simulink model "test03"  (R2021a)
settings: Solver=VariableStepAuto  StartTime=0.0  StopTime=10  RelTol=1e-3
values from neighbouring files (symbols this model uses):
  cic = climate_ic    [test03_script.m]
  params = climate_p    [test03_script.m]
libraries: HORTISIM x8
settings Model: Creator=djoroya  LastModifiedBy=djoroya
settings DebuggingCC: UnconnectedInputMsg=none  UnconnectedOutputMsg=none  UnconnectedLineMsg=none

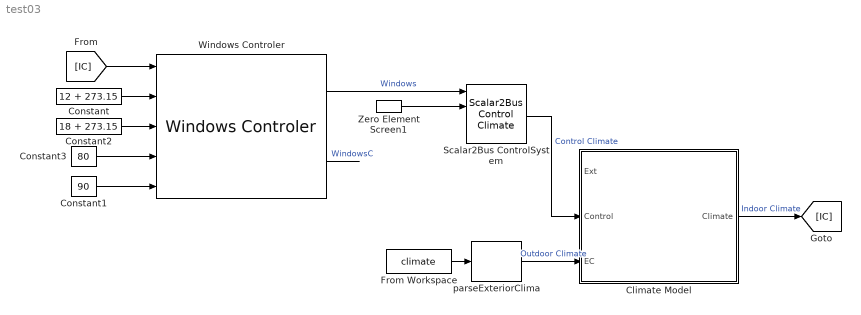
== system test03 ==
  Climate Model : Subsystem  AncestorBlock=HORTISIM/Climate/Models/Climate Model  mask{params=params, x0=cic}
      mask Display: image('$imagefile'); % Use "Edit Image" on toolstrip to change.
  Constant : Constant  Value=12 + 273.15
  Constant1 : Constant  Value=90
  Constant2 : Constant  Value=18 + 273.15
  Constant3 : Constant  Value=80
  From Workspace : FromWorkspace  VariableName=climate
  Scalar2Bus ControlSystem : HORTISIM/Other  Functions/Scalar2Bus  Control Climate  SystemSampleTime=-1  VariantActivationTime=update diagram  Latency=0  AutoFrameSizeCalculation=off
      settings: SourceProductName=Horti Simulator
  Windows Controler : HORTISIM/Climate/Controls/Windows Controler  params=win_p
      settings: SourceProductName=Horti Simulator
  Zero Element Screen1 : HORTISIM/Other  Functions/Zero Element Screen  SystemSampleTime=-1  VariantActivationTime=update diagram  Latency=0  AutoFrameSizeCalculation=off
      settings: SourceProductName=Horti Simulator
  parseExteriorClima : HORTISIM/Other  Functions/parseExteriorClima  SystemSampleTime=-1  VariantActivationTime=update diagram  Latency=0  AutoFrameSizeCalculation=off
      settings: SourceProductName=Horti Simulator
  wires:
  From Workspace/1 -> parseExteriorClima/1
  parseExteriorClima/1 -> Climate Model/3(EC)  "Outdoor Climate"
  Climate Model/1(Climate) -> [IC]  "Indoor Climate"
  Scalar2Bus ControlSystem/1 -> Climate Model/2(Control)  "Control Climate"
  Windows Controler/1 -> Scalar2Bus ControlSystem/1  "Windows"
  [IC] -> Windows Controler/1
  Constant/1 -> Windows Controler/2
  Constant2/1 -> Windows Controler/3
  Constant3/1 -> Windows Controler/4
  Constant1/1 -> Windows Controler/5
  Windows Controler/2 -> ?  "WindowsC"
  Zero Element Screen1/1 -> Scalar2Bus ControlSystem/2

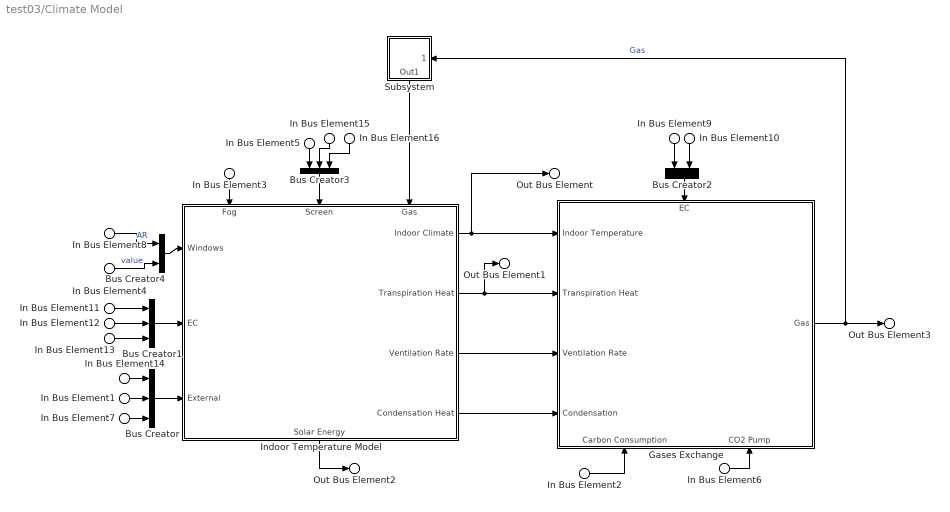
== system test03/Climate Model ==
  In Bus Element14 : Inport  PortName=Ext  Element=QT
  In Bus Element1 : Inport  PortName=Ext  Element=QV
  In Bus Element2 : Inport  PortName=Ext  Element=CC
  In Bus Element7 : Inport  PortName=Ext  Element=A
  In Bus Element3 : Inport  Port=2  PortName=Control  Element=Fog
  In Bus Element5 : Inport  Port=2  PortName=Control  Element=Screen.gamma_max
  In Bus Element15 : Inport  Port=2  PortName=Control  Element=Screen.value
  In Bus Element16 : Inport  Port=2  PortName=Control  Element=Screen.beta
  In Bus Element6 : Inport  Port=2  PortName=Control  Element=CO2
  In Bus Element8 : Inport  Port=2  PortName=Control  Element=Windows.AR
  In Bus Element4 : Inport  Port=2  PortName=Control  Element=Windows.value
  In Bus Element9 : Inport  Port=3  PortName=EC  Element=HR
  In Bus Element10 : Inport  Port=3  PortName=EC  Element=Temp
  In Bus Element11 : Inport  Port=3  PortName=EC  Element=Temp
  In Bus Element12 : Inport  Port=3  PortName=EC  Element=Rad
  In Bus Element13 : Inport  Port=3  PortName=EC  Element=Wind
  Bus Creator : BusCreator  Inputs=3
  Bus Creator1 : BusCreator  Inputs=3
  Bus Creator2 : BusCreator  Inputs=2
  Bus Creator3 : BusCreator  Inputs=3
  Bus Creator4 : BusCreator  Inputs=2
  Gases Exchange : Subsystem
      settings: PortSchema="{\"entries\":[{\"content\":{\"sides\":[{\"content\":{\"connectorIds\":[\"In1\",\"In2\",\"In3\",\"In4\"]},\"type\":\"ConnectorPlacement.EquallySpacedRectSide\",\"uuid\":\"550da9a1-5f22-4db3-9ee3-e3750278f626\"},{\"content\":{\"connectorIds\":[\"Out1\"],\"side\":\"RIGHT\"},\"type\":\"ConnectorPlacement.EquallySpacedRectSide\",\"uuid\":\"cf559ec0-337d-42e7-96bb-a49ff9e682f6\"},{\"content\":{\"connectorIds\":[\"In5\"],\"side\":\"TOP\"},\"type\":\"ConnectorPlacement.EquallySpacedRectSide\",\"uuid\":\"d9874986-c35c-443c-9325-7a886074565b\"},{\"content\":{\"connectorIds\":[\"In6\",\"In7\"],\"side\":\"BOTTOM\"},\"type\":\"ConnectorPlacement.EquallySpacedRectSide\",\"uuid\":\"7f205c84-db2c-43a4-94ce-a6d2142a4e50\"}]},\"type\":\"ConnectorPlacement.EquallySpacedConnector\",\"uuid\":\"56c5cbc1-f580-43fc-9d79-62500ce9be4b\"}],\"packageUris\":[\"http://schema.mathworks.com/mf0/Connector/R2020b\"],\"version\":\"1.0\"}"
  Indoor Temperature Model : Subsystem
      settings: PortSchema="{\"entries\":[{\"content\":{\"sides\":[{\"content\":{\"connectorIds\":[\"In1\",\"In2\",\"In3\"]},\"type\":\"ConnectorPlacement.EquallySpacedRectSide\",\"uuid\":\"402556d7-b277-4cb3-8556-883bae99c69c\"},{\"content\":{\"connectorIds\":[\"Out1\",\"Out2\",\"Out3\",\"Out4\"],\"side\":\"RIGHT\"},\"type\":\"ConnectorPlacement.EquallySpacedRectSide\",\"uuid\":\"e8ec9f82-8759-4d98-a5e5-ef4db996ec8c\"},{\"content\":{\"connectorIds\":[\"In4\",\"In5\",\"In6\"],\"side\":\"TOP\"},\"type\":\"ConnectorPlacement.EquallySpacedRectSide\",\"uuid\":\"99d33cea-a089-4bcb-9505-68914c63f152\"},{\"content\":{\"connectorIds\":[\"Out5\"],\"side\":\"BOTTOM\"},\"type\":\"ConnectorPlacement.EquallySpacedRectSide\",\"uuid\":\"61ead6b3-0464-47f9-9f23-19f86056b325\"}]},\"type\":\"ConnectorPlacement.EquallySpacedConnector\",\"uuid\":\"a07dfd2f-7b40-4439-87f5-f093ac984b26\"}],\"packageUris\":[\"http://schema.mathworks.com/mf0/Connector/R2020b\"],\"version\":\"1.0\"}"
  Subsystem : Subsystem
      settings: PortSchema="{\"entries\":[{\"content\":{\"sides\":[{\"content\":{\"connectorIds\":[]},\"type\":\"ConnectorPlacement.EquallySpacedRectSide\",\"uuid\":\"35868875-f783-4ad4-af7a-8ba6d23e35d0\"},{\"content\":{\"connectorIds\":[\"Out1\"],\"side\":\"RIGHT\"},\"type\":\"ConnectorPlacement.EquallySpacedRectSide\",\"uuid\":\"2025d12d-e021-4399-bfe6-d7037c727539\"},{\"content\":{\"connectorIds\":[],\"side\":\"TOP\"},\"type\":\"ConnectorPlacement.EquallySpacedRectSide\",\"uuid\":\"3e424627-322e-4117-9014-21364a52cbdc\"},{\"content\":{\"connectorIds\":[\"In1\"],\"side\":\"BOTTOM\"},\"type\":\"ConnectorPlacement.EquallySpacedRectSide\",\"uuid\":\"db7a2526-7ee4-413d-8e1d-de852bb4cdfb\"}]},\"type\":\"ConnectorPlacement.EquallySpacedConnector\",\"uuid\":\"c6534136-4261-4144-9645-4fbbe9dd779a\"}],\"packageUris\":[\"http://schema.mathworks.com/mf0/Connector/R2020b\"],\"version\":\"1.0\"}"
  Out Bus Element : Outport  PortName=Climate  Element=Temp
  Out Bus Element1 : Outport  PortName=Climate  Element=QT
  Out Bus Element2 : Outport  PortName=Climate  Element=QS
  Out Bus Element3 : Outport  PortName=Climate  Element=Gas
  wires:
  In Bus Element7/1 -> Bus Creator/3
  Bus Creator/1 -> Indoor Temperature Model/3(External)
  In Bus Element14/1 -> Bus Creator/1
  In Bus Element1/1 -> Bus Creator/2
  In Bus Element10/1 -> Bus Creator2/2
  In Bus Element9/1 -> Bus Creator2/1
  Bus Creator2/1 -> Gases Exchange/5(EC)
  Bus Creator1/1 -> Indoor Temperature Model/2(EC)
  In Bus Element11/1 -> Bus Creator1/1
  In Bus Element13/1 -> Bus Creator1/3
  In Bus Element12/1 -> Bus Creator1/2
  In Bus Element6/1 -> Gases Exchange/7(CO2 Pump)
  In Bus Element3/1 -> Indoor Temperature Model/4(Fog)
  Indoor Temperature Model/5(Solar Energy) -> Out Bus Element2/1
  Indoor Temperature Model/2(Transpiration Heat) -> Out Bus Element1/1, Gases Exchange/2(Transpiration Heat)
  Indoor Temperature Model/1(Indoor Climate) -> Gases Exchange/1(Indoor Temperature), Out Bus Element/1
  Indoor Temperature Model/3(Ventilation Rate) -> Gases Exchange/3(Ventilation Rate)
  Indoor Temperature Model/4(Condensation Heat) -> Gases Exchange/4(Condensation)
  In Bus Element2/1 -> Gases Exchange/6(Carbon Consumption)
  Gases Exchange/1(" Gas") -> Subsystem/1(Gas), Out Bus Element3/1  "Gas"
  In Bus Element4/1 -> Bus Creator4/2  "value"
  In Bus Element8/1 -> Bus Creator4/1  "AR"
  Bus Creator4/1 -> Indoor Temperature Model/1(Windows)
  Subsystem/1(Out1) -> Indoor Temperature Model/6(Gas)
  Bus Creator3/1 -> Indoor Temperature Model/5(Screen)
  In Bus Element5/1 -> Bus Creator3/1
  In Bus Element15/1 -> Bus Creator3/2
  In Bus Element16/1 -> Bus Creator3/3

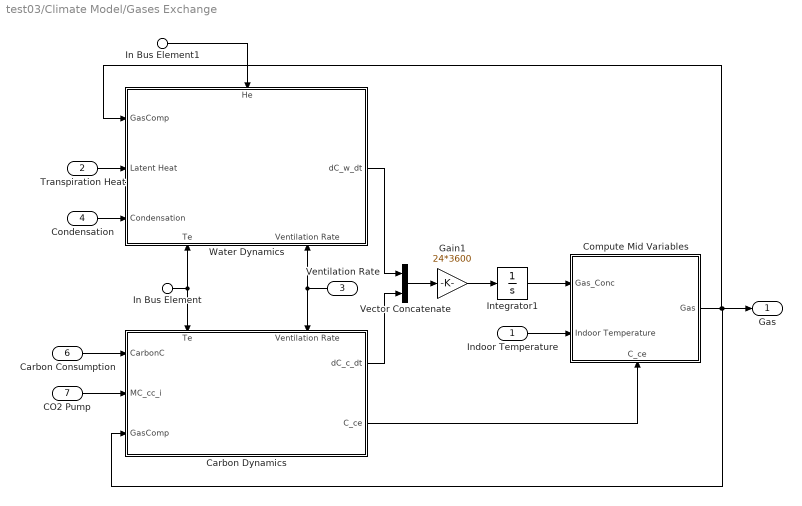
== system test03/Climate Model/Gases Exchange ==
  Indoor Temperature : Inport
  Transpiration Heat : Inport  Port=2
  Ventilation Rate : Inport  Port=3
  Condensation : Inport  Port=4
  In Bus Element : Inport  Port=5  PortName=EC  Element=Temp
  In Bus Element1 : Inport  Port=5  PortName=EC  Element=HR
  Carbon Consumption : Inport  Port=6
  CO2 Pump : Inport  Port=7
  Carbon Dynamics : Subsystem
      settings: PortSchema="{\"entries\":[{\"content\":{\"sides\":[{\"content\":{\"connectorIds\":[\"In1\",\"In2\",\"In3\"]},\"type\":\"ConnectorPlacement.EquallySpacedRectSide\",\"uuid\":\"ce6da3e3-21f1-4394-8848-c3b9ed37cfe4\"},{\"content\":{\"connectorIds\":[\"Out1\",\"Out2\"],\"side\":\"RIGHT\"},\"type\":\"ConnectorPlacement.EquallySpacedRectSide\",\"uuid\":\"ff9d1dc7-ad1d-4f02-8424-55a857bc099f\"},{\"content\":{\"connectorIds\":[\"In4\",\"In5\"],\"side\":\"TOP\"},\"type\":\"ConnectorPlacement.EquallySpacedRectSide\",\"uuid\":\"728a06d8-4ce2-49f0-80dc-b6302b266d7a\"}]},\"type\":\"ConnectorPlacement.EquallySpacedConnector\",\"uuid\":\"a07ea8b7-add0-4d37-8d5e-856da5f5b640\"}],\"packageUris\":[\"http://schema.mathworks.com/mf0/Connector/R2020b\"],\"version\":\"1.0\"}"
  Compute Mid Variables : Subsystem
      settings: PortSchema="{\"entries\":[{\"content\":{\"sides\":[{\"content\":{\"connectorIds\":[\"In1\",\"In2\"]},\"type\":\"ConnectorPlacement.EquallySpacedRectSide\",\"uuid\":\"c9e251e2-f19d-4856-b15c-3b9f1eb64f83\"},{\"content\":{\"connectorIds\":[\"Out1\"],\"side\":\"RIGHT\"},\"type\":\"ConnectorPlacement.EquallySpacedRectSide\",\"uuid\":\"10734817-c937-42fb-8ae5-9505620c6f0f\"},{\"content\":{\"connectorIds\":[],\"side\":\"TOP\"},\"type\":\"ConnectorPlacement.EquallySpacedRectSide\",\"uuid\":\"8c056440-d8bf-4ff4-85aa-0f6a5eb7f23f\"},{\"content\":{\"connectorIds\":[\"In3\"],\"side\":\"BOTTOM\"},\"type\":\"ConnectorPlacement.EquallySpacedRectSide\",\"uuid\":\"fc2511c5-58d6-455e-9438-4abf6bda86a2\"}]},\"type\":\"ConnectorPlacement.EquallySpacedConnector\",\"uuid\":\"13e72cfa-9d8f-4756-adac-f24fb0238c2a\"}],\"packageUris\":[\"http://schema.mathworks.com/mf0/Connector/R2020b\"],\"version\":\"1.0\"}"
  Gain1 : Gain  Gain=24*3600
  Integrator1 : Integrator  InitialCondition=x0.G0  AbsoluteTolerance=1e-5
  Vector Concatenate : Concatenate
  Water Dynamics : Subsystem
      settings: PortSchema="{\"entries\":[{\"content\":{\"sides\":[{\"content\":{\"connectorIds\":[\"In1\",\"In2\",\"In3\"]},\"type\":\"ConnectorPlacement.EquallySpacedRectSide\",\"uuid\":\"ce6da3e3-21f1-4394-8848-c3b9ed37cfe4\"},{\"content\":{\"connectorIds\":[\"Out1\"],\"side\":\"RIGHT\"},\"type\":\"ConnectorPlacement.EquallySpacedRectSide\",\"uuid\":\"ff9d1dc7-ad1d-4f02-8424-55a857bc099f\"},{\"content\":{\"connectorIds\":[\"In4\"],\"side\":\"TOP\"},\"type\":\"ConnectorPlacement.EquallySpacedRectSide\",\"uuid\":\"728a06d8-4ce2-49f0-80dc-b6302b266d7a\"},{\"content\":{\"connectorIds\":[\"In5\",\"In6\"],\"side\":\"BOTTOM\"},\"type\":\"ConnectorPlacement.EquallySpacedRectSide\",\"uuid\":\"cc1d9c53-b6c6-41b0-b878-c109c9de6d5f\"}]},\"type\":\"ConnectorPlacement.EquallySpacedConnector\",\"uuid\":\"a07ea8b7-add0-4d37-8d5e-856da5f5b640\"}],\"packageUris\":[\"http://schema.mathworks.com/mf0/Connector/R2020b\"],\"version\":\"1.0\"}"
  " Gas" : Outport
  wires:
  Carbon Dynamics/2(C_ce) -> Compute Mid Variables/3(C_ce)
  In Bus Element1/1 -> Water Dynamics/4(He)
  In Bus Element/1 -> Water Dynamics/5(Te), Carbon Dynamics/4(Te)
  CO2 Pump/1 -> Carbon Dynamics/2(MC_cc_i)
  Condensation/1 -> Water Dynamics/3(Condensation)
  Compute Mid Variables/1(Gas) -> " Gas"/1, Carbon Dynamics/3(GasComp), Water Dynamics/1(GasComp)
  Indoor Temperature/1 -> Compute Mid Variables/2(Indoor Temperature)
  Ventilation Rate/1 -> Water Dynamics/6(Ventilation Rate), Carbon Dynamics/5(Ventilation Rate)
  Carbon Dynamics/1(dC_c_dt) -> Vector Concatenate/2
  Carbon Consumption/1 -> Carbon Dynamics/1(CarbonC)
  Water Dynamics/1(dC_w_dt) -> Vector Concatenate/1
  Transpiration Heat/1 -> Water Dynamics/2(Latent Heat)
  Integrator1/1 -> Compute Mid Variables/1(Gas_Conc)
  Vector Concatenate/1 -> Gain1/1
  Gain1/1 -> Integrator1/1

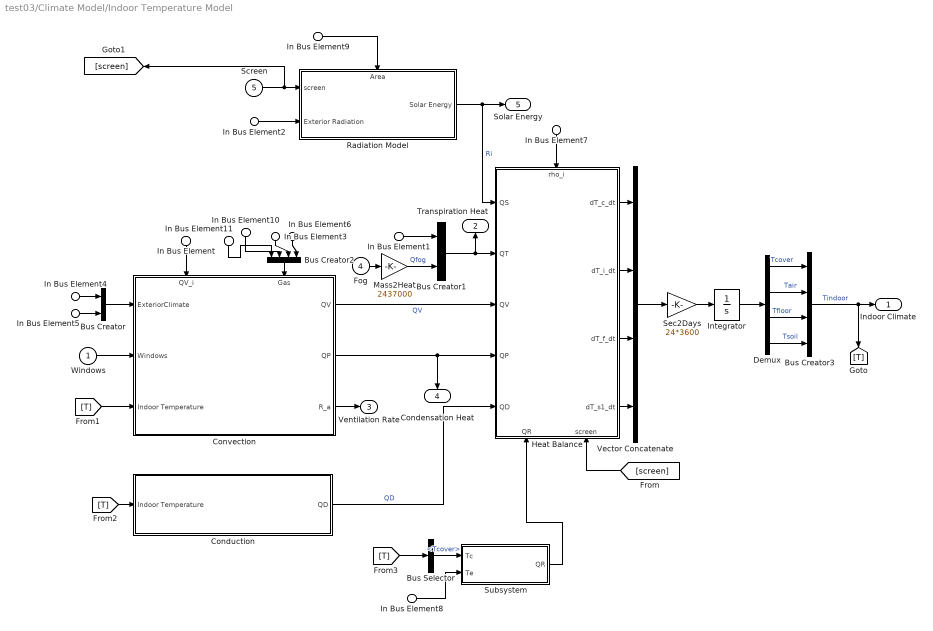
== system test03/Climate Model/Indoor Temperature Model ==
  Windows : Inport
  In Bus Element2 : Inport  Port=2  PortName=EC  Element=Rad
  In Bus Element4 : Inport  Port=2  PortName=EC  Element=Temp
  In Bus Element8 : Inport  Port=2  PortName=EC  Element=Temp
  In Bus Element5 : Inport  Port=2  PortName=EC  Element=Wind
  In Bus Element : Inport  Port=3  PortName=External  Element=QV
  In Bus Element1 : Inport  Port=3  PortName=External  Element=QT
  In Bus Element9 : Inport  Port=3  PortName=External  Element=A
  Fog : Inport  Port=4
  Screen : Inport  Port=5
  In Bus Element3 : Inport  Port=6  PortName=Gas  Element=C_w
  In Bus Element6 : Inport  Port=6  PortName=Gas  Element=rho_i
  In Bus Element7 : Inport  Port=6  PortName=Gas  Element=rho_i
  In Bus Element10 : Inport  Port=6  PortName=Gas  Element=C_w_sat_T_c
  In Bus Element11 : Inport  Port=6  PortName=Gas  Element=C_w_sat_T_f
  Bus Creator : BusCreator  Inputs=2
  Bus Creator1 : BusCreator  Inputs=2
  Bus Creator2 : BusCreator  Inputs=4
  Bus Creator3 : BusCreator  Inputs=4
  Bus Selector : BusSelector  OutputSignals=Tcover
  Conduction : Subsystem
  Convection : Subsystem
      settings: PortSchema="{\"entries\":[{\"content\":{\"sides\":[{\"content\":{\"connectorIds\":[\"In1\",\"In2\",\"In3\"]},\"type\":\"ConnectorPlacement.EquallySpacedRectSide\",\"uuid\":\"3a7e199a-659d-4634-89e1-ef85cb7ed502\"},{\"content\":{\"connectorIds\":[\"Out1\",\"Out2\",\"Out3\"],\"side\":\"RIGHT\"},\"type\":\"ConnectorPlacement.EquallySpacedRectSide\",\"uuid\":\"10ed7806-8be5-4e88-a0ca-6abfb5c9ab8d\"},{\"content\":{\"connectorIds\":[\"In4\",\"In5\"],\"side\":\"TOP\"},\"type\":\"ConnectorPlacement.EquallySpacedRectSide\",\"uuid\":\"907defe4-ff8f-4a74-ba27-620529c27b74\"},{\"content\":{\"connectorIds\":[],\"side\":\"BOTTOM\"},\"type\":\"ConnectorPlacement.EquallySpacedRectSide\",\"uuid\":\"397bdb42-e8ee-4be9-8569-3130f6cbf999\"}]},\"type\":\"ConnectorPlacement.EquallySpacedConnector\",\"uuid\":\"f437f85f-61b6-4f41-a544-29e333cf1086\"}],\"packageUris\":[\"http://schema.mathworks.com/mf0/Connector/R2020b\"],\"version\":\"1.0\"}"
  Demux : Demux
  Heat Balance : Subsystem
      settings: PortSchema="{\"entries\":[{\"content\":{\"sides\":[{\"content\":{\"connectorIds\":[\"In1\",\"In2\",\"In3\",\"In4\",\"In5\"]},\"type\":\"ConnectorPlacement.EquallySpacedRectSide\",\"uuid\":\"ccfbb954-e9e7-4841-9dc1-a760315eb250\"},{\"content\":{\"connectorIds\":[\"Out1\",\"Out2\",\"Out3\",\"Out4\"],\"side\":\"RIGHT\"},\"type\":\"ConnectorPlacement.EquallySpacedRectSide\",\"uuid\":\"e9754eb2-54ce-43cf-bf33-7cf2f1345c42\"},{\"content\":{\"connectorIds\":[\"In6\"],\"side\":\"TOP\"},\"type\":\"ConnectorPlacement.EquallySpacedRectSide\",\"uuid\":\"6ccd5de1-b6bb-47c5-ac6c-9382e354fee6\"},{\"content\":{\"connectorIds\":[\"In7\",\"In8\"],\"side\":\"BOTTOM\"},\"type\":\"ConnectorPlacement.EquallySpacedRectSide\",\"uuid\":\"dba41702-708c-4231-8998-8d54661f4881\"}]},\"type\":\"ConnectorPlacement.EquallySpacedConnector\",\"uuid\":\"31920c9d-5e0f-4503-9ddd-ce99d792a3e0\"}],\"packageUris\":[\"http://schema.mathworks.com/mf0/Connector/R2020b\"],\"version\":\"1.0\"}"
  Integrator : Integrator  InitialCondition=x0.T0  AbsoluteTolerance=0.01
  Mass2Heat : Gain  Gain=2437000
  Radiation Model : Subsystem
      settings: PortSchema="{\"entries\":[{\"content\":{\"sides\":[{\"content\":{\"connectorIds\":[\"In1\",\"In2\"]},\"type\":\"ConnectorPlacement.EquallySpacedRectSide\",\"uuid\":\"cb5a2538-07d5-409a-bc47-ac7157db0ef4\"},{\"content\":{\"connectorIds\":[\"Out1\"],\"side\":\"RIGHT\"},\"type\":\"ConnectorPlacement.EquallySpacedRectSide\",\"uuid\":\"7dfe2e6f-8ee6-45c0-8502-080571e1b483\"},{\"content\":{\"connectorIds\":[\"In3\"],\"side\":\"TOP\"},\"type\":\"ConnectorPlacement.EquallySpacedRectSide\",\"uuid\":\"52df64bb-9cf1-44e4-8c24-fa6c372d73f1\"}]},\"type\":\"ConnectorPlacement.EquallySpacedConnector\",\"uuid\":\"b803895f-b114-4368-b273-36a7794022b5\"}],\"packageUris\":[\"http://schema.mathworks.com/mf0/Connector/R2020b\"],\"version\":\"1.0\"}"
  Sec2Days : Gain  Gain=24*3600
  Subsystem : Subsystem
  Vector Concatenate : Concatenate  NumInputs=4
  Indoor Climate : Outport
  Transpiration Heat : Outport  Port=2
  Ventilation Rate : Outport  Port=3
  Condensation Heat : Outport  Port=4
  Solar Energy : Outport  Port=5
  wires:
  In Bus Element11/1 -> Bus Creator2/1
  In Bus Element10/1 -> Bus Creator2/2
  In Bus Element9/1 -> Radiation Model/3(Area)
  Subsystem/1(QR) -> Heat Balance/7(QR)
  Bus Selector/1 -> Subsystem/1(Tc)  "<Tcover>"
  [T] -> Bus Selector/1
  In Bus Element8/1 -> Subsystem/2(Te)
  Integrator/1 -> Demux/1
  Demux/1 -> Bus Creator3/1  "Tcover"
  Demux/2 -> Bus Creator3/2  "Tair"
  Demux/3 -> Bus Creator3/3  "Tfloor"
  Demux/4 -> Bus Creator3/4  "Tsoil"
  Bus Creator3/1 -> Indoor Climate/1, [T]  "Tindoor"
  In Bus Element/1 -> Convection/4(QV_i)
  In Bus Element6/1 -> Bus Creator2/4
  In Bus Element3/1 -> Bus Creator2/3
  Bus Creator2/1 -> Convection/5(Gas)
  Bus Creator1/1 -> Transpiration Heat/1, Heat Balance/2(QT)
  In Bus Element1/1 -> Bus Creator1/1
  Mass2Heat/1 -> Bus Creator1/2  "Qfog"
  Fog/1 -> Mass2Heat/1
  In Bus Element5/1 -> Bus Creator/2
  In Bus Element4/1 -> Bus Creator/1
  Screen/1 -> [screen], Radiation Model/1(screen)
  Bus Creator/1 -> Convection/1(ExteriorClimate)
  Radiation Model/1("Solar Energy  ") -> Heat Balance/1(QS), Solar Energy/1  "Ri"
  In Bus Element2/1 -> Radiation Model/2(Exterior Radiation)
  Windows/1 -> Convection/2(Windows)
  Convection/2(QP) -> Heat Balance/4(QP), Condensation Heat/1
  In Bus Element7/1 -> Heat Balance/6(rho_i)
  [T] -> Conduction/1(Indoor Temperature)
  [T] -> Convection/3(Indoor Temperature)
  Heat Balance/1(dT_c_dt) -> Vector Concatenate/1
  Heat Balance/4(dT_s1_dt) -> Vector Concatenate/4
  Heat Balance/3(dT_f_dt) -> Vector Concatenate/3
  Heat Balance/2(dT_i_dt) -> Vector Concatenate/2
  Conduction/1(QD) -> Heat Balance/5(QD)  "QD"
  Convection/1(QV) -> Heat Balance/3(QV)  "QV"
  Convection/3(R_a) -> Ventilation Rate/1
  Sec2Days/1 -> Integrator/1
  Vector Concatenate/1 -> Sec2Days/1
  [screen] -> Heat Balance/8(screen)

== system test03/Climate Model/Subsystem ==
  Gas : Inport
  Bus Creator3 : BusCreator  Inputs=4
  Bus Selector : BusSelector  OutputSignals=C_w,rho_i,C_w_sat_T_c,C_w_sat_T_f
  Out1 : Outport
  wires:
  Gas/1 -> Bus Selector/1
  Bus Selector/4 -> Bus Creator3/4  "<C_w_sat_T_f>"
  Bus Selector/2 -> Bus Creator3/2  "<rho_i>"
  Bus Selector/1 -> Bus Creator3/1  "<C_w>"
  Bus Creator3/1 -> Out1/1
  Bus Selector/3 -> Bus Creator3/3  "<C_w_sat_T_c>"

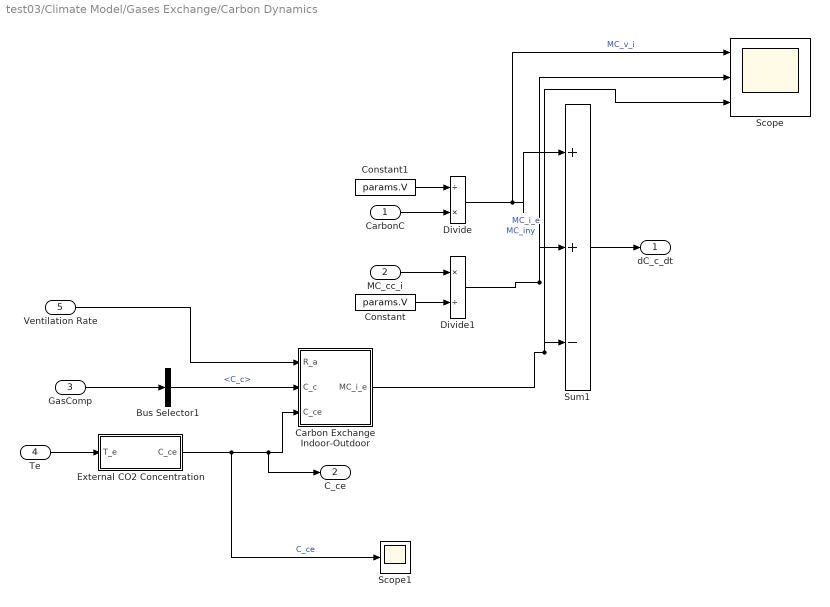
== system test03/Climate Model/Gases Exchange/Carbon Dynamics ==
  CarbonC : Inport
  MC_cc_i : Inport  Port=2
  GasComp : Inport  Port=3
  Te : Inport  Port=4
  Ventilation Rate : Inport  Port=5
  Bus Selector1 : BusSelector  OutputSignals=C_c
  Carbon Exchange Indoor-Outdoor : Subsystem
  Constant : Constant  Value=params.V
  Constant1 : Constant  Value=params.V
  Divide : Product  Inputs=/*
  Divide1 : Product  Inputs=*/
  External CO2 Concentration : Subsystem
  Scope : Scope  NumInputPorts=3
  Scope1 : Scope
  Sum1 : Sum  Inputs=|++-
  dC_c_dt : Outport
  C_ce : Outport  Port=2
  wires:
  Constant1/1 -> Divide/1
  Constant/1 -> Divide1/2
  Te/1 -> External CO2 Concentration/1(T_e)
  Sum1/1 -> dC_c_dt/1
  Carbon Exchange Indoor-Outdoor/1(MC_i_e) -> Sum1/3, Scope/3  "MC_i_e"
  Divide1/1 -> Sum1/2, Scope/2  "MC_iny"
  Divide/1 -> Sum1/1, Scope/1  "MC_v_i"
  MC_cc_i/1 -> Divide1/1
  External CO2 Concentration/1(C_ce) -> Carbon Exchange Indoor-Outdoor/3(C_ce), C_ce/1, Scope1/1  "C_ce"
  Bus Selector1/1 -> Carbon Exchange Indoor-Outdoor/2(C_c)  "<C_c>"
  GasComp/1 -> Bus Selector1/1
  CarbonC/1 -> Divide/2
  Ventilation Rate/1 -> Carbon Exchange Indoor-Outdoor/1(R_a)

== system test03/Climate Model/Gases Exchange/Compute Mid Variables ==
  Gas_Conc : Inport
  Indoor Temperature : Inport  Port=2
  C_ce : Inport  Port=3
  Bus Creator : BusCreator  Inputs=12
  Constant : Constant  Value=params.int_air_speed
  Demux : Demux  Outputs=2
  Subsystem : Subsystem
  Gas : Outport
  wires:
  C_ce/1 -> Bus Creator/12  "C_ce"
  Subsystem/8(xH_sat) -> Bus Creator/11  "Xh_sat"
  Subsystem/7(p_a) -> Bus Creator/10  "p_a"
  Subsystem/5(C_w_sat_T_f) -> Bus Creator/8  "C_w_sat_T_f"
  Subsystem/4(C_w_sat_T_c) -> Bus Creator/7  "C_w_sat_T_c"
  Subsystem/6(xH) -> Bus Creator/9  "Xh"
  Demux/1 -> Bus Creator/2  "C_w"
  Constant/1 -> Bus Creator/1  "air_speed"
  Indoor Temperature/1 -> Subsystem/2(IndoorTemp)
  Demux/2 -> Bus Creator/3  "C_c"
  Subsystem/3(HRInt) -> Bus Creator/6  "HRInt"
  Subsystem/2(C_c_ppm) -> Bus Creator/5  "C_c_ppm"
  Subsystem/1(rho_i) -> Bus Creator/4  "rho_i"
  Bus Creator/1 -> Gas/1  "Gas"
  Gas_Conc/1 -> Subsystem/1(Gas_Conc), Demux/1

== system test03/Climate Model/Gases Exchange/Water Dynamics ==
  GasComp : Inport
  Latent Heat : Inport  Port=2
  Condensation : Inport  Port=3
  He : Inport  Port=4
  Te : Inport  Port=5
  Ventilation Rate : Inport  Port=6
  Bus Selector : BusSelector  OutputSignals=QT,Qfog
  Bus Selector1 : BusSelector  OutputSignals=C_w
  Bus Selector2 : BusSelector  OutputSignals=QP_i_c,QP_i_f
  Minus : Sum  Inputs=+-
  Product : Product
  Subsystem : Subsystem
  Vapor Mass Balance : Subsystem
  dC_w_dt : Outport
  wires:
  Vapor Mass Balance/1(dC_w_dt) -> dC_w_dt/1
  Bus Selector2/2 -> Vapor Mass Balance/5(<QP_i_f>)  "<QP_i_f>"
  Bus Selector2/1 -> Vapor Mass Balance/4(<QP_i_c>)  "<QP_i_c>"
  Product/1 -> Vapor Mass Balance/3(MW_i_e)
  Bus Selector/2 -> Vapor Mass Balance/2(<Qfog>)  "<Qfog>"
  Subsystem/1(C_w_Te) -> Minus/2
  He/1 -> Subsystem/2(<Exterior Humidity>)
  Te/1 -> Subsystem/1(<Temperature>)
  Minus/1 -> Product/2
  Condensation/1 -> Bus Selector2/1
  Bus Selector1/1 -> Minus/1  "<C_w>"
  GasComp/1 -> Bus Selector1/1
  Bus Selector/1 -> Vapor Mass Balance/1(<QT_v_i>)  "<QT>"
  Latent Heat/1 -> Bus Selector/1
  Ventilation Rate/1 -> Product/1

== system test03/Climate Model/Indoor Temperature Model/Conduction ==
  Indoor Temperature : Inport
  Bus Creator : BusCreator  Inputs=2
  Bus Selector : BusSelector  OutputSignals=Tfloor,Tsoil
  Conduction : MATLAB Function  TreatAsAtomicUnit=on
  Constant : Constant  Value=params.A_f
  Constant1 : Constant  Value=params.lam_s
  Constant2 : Constant  Value=params.l_s
  Constant3 : Constant  Value=params.T_ss
  QD : Outport
  wires:
  Constant/1 -> Conduction/3(A_f)
  Constant1/1 -> Conduction/4(lam_s)
  Constant2/1 -> Conduction/5(l_s)
  Constant3/1 -> Conduction/6(T_ss)
  Bus Selector/1 -> Conduction/1(T_f)  "<Tfloor>"
  Bus Selector/2 -> Conduction/2(T_s1)  "<Tsoil>"
  Indoor Temperature/1 -> Bus Selector/1
  Bus Creator/1 -> QD/1
  Conduction/2(QD_s12) -> Bus Creator/2
  Conduction/1(QD_sf1) -> Bus Creator/1

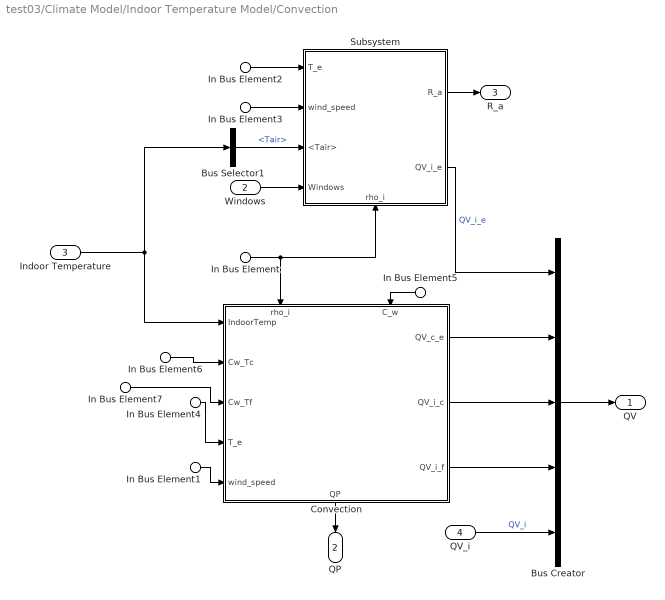
== system test03/Climate Model/Indoor Temperature Model/Convection ==
  In Bus Element2 : Inport  PortName=ExteriorClimate  Element=Temp
  In Bus Element4 : Inport  PortName=ExteriorClimate  Element=Temp
  In Bus Element1 : Inport  PortName=ExteriorClimate  Element=Wind
  In Bus Element3 : Inport  PortName=ExteriorClimate  Element=Wind
  Windows : Inport  Port=2
  Indoor Temperature : Inport  Port=3
  QV_i : Inport  Port=4
  In Bus Element : Inport  Port=5  PortName=Gas  Element=rho_i
  In Bus Element5 : Inport  Port=5  PortName=Gas  Element=C_w
  In Bus Element6 : Inport  Port=5  PortName=Gas  Element=C_w_sat_T_c
  In Bus Element7 : Inport  Port=5  PortName=Gas  Element=C_w_sat_T_f
  Bus Creator : BusCreator  Inputs=5
  Bus Selector1 : BusSelector  OutputSignals=Tair
  Convection : Subsystem
      settings: PortSchema="{\"entries\":[{\"content\":{\"sides\":[{\"content\":{\"connectorIds\":[\"In1\",\"In2\",\"In3\",\"In4\",\"In5\"]},\"type\":\"ConnectorPlacement.EquallySpacedRectSide\",\"uuid\":\"490685c0-4e11-426f-bb8f-3f4d655c5ac7\"},{\"content\":{\"connectorIds\":[\"Out1\",\"Out2\",\"Out3\"],\"side\":\"RIGHT\"},\"type\":\"ConnectorPlacement.EquallySpacedRectSide\",\"uuid\":\"d4812e49-5d44-4dbe-a973-0d0765960a30\"},{\"content\":{\"connectorIds\":[\"In6\",\"In7\"],\"side\":\"TOP\"},\"type\":\"ConnectorPlacement.EquallySpacedRectSide\",\"uuid\":\"13a56147-4397-4d7e-8a08-f4127ff1f422\"},{\"content\":{\"connectorIds\":[\"Out4\"],\"side\":\"BOTTOM\"},\"type\":\"ConnectorPlacement.EquallySpacedRectSide\",\"uuid\":\"3700cf61-bbb7-4a7e-bcc8-2fc27ab64caf\"}]},\"type\":\"ConnectorPlacement.EquallySpacedConnector\",\"uuid\":\"ceadb976-1cc2-4430-962a-7e8db98fda5f\"}],\"packageUris\":[\"http://schema.mathworks.com/mf0/Connector/R2020b\"],\"version\":\"1.0\"}"
  Subsystem : Subsystem
      settings: PortSchema="{\"entries\":[{\"content\":{\"sides\":[{\"content\":{\"connectorIds\":[\"In1\",\"In2\",\"In3\",\"In4\"]},\"type\":\"ConnectorPlacement.EquallySpacedRectSide\",\"uuid\":\"b628b76c-815c-4d2d-bf8b-9241abf78a18\"},{\"content\":{\"connectorIds\":[\"Out1\",\"Out2\"],\"side\":\"RIGHT\"},\"type\":\"ConnectorPlacement.EquallySpacedRectSide\",\"uuid\":\"d01161a9-1f84-445a-b084-f8cb6d6fe506\"},{\"content\":{\"connectorIds\":[],\"side\":\"TOP\"},\"type\":\"ConnectorPlacement.EquallySpacedRectSide\",\"uuid\":\"e7ae8035-b56b-4ea0-80c9-470a91dd5096\"},{\"content\":{\"connectorIds\":[\"In5\"],\"side\":\"BOTTOM\"},\"type\":\"ConnectorPlacement.EquallySpacedRectSide\",\"uuid\":\"28955d4e-ecf1-4383-b712-07fa8a44f693\"}]},\"type\":\"ConnectorPlacement.EquallySpacedConnector\",\"uuid\":\"e2661f4d-c009-47a9-b3ca-7a17d9ffa541\"}],\"packageUris\":[\"http://schema.mathworks.com/mf0/Connector/R2020b\"],\"version\":\"1.0\"}"
  QV : Outport  PortDimensions=5
  QP : Outport  Port=2
  R_a : Outport  Port=3
  wires:
  In Bus Element7/1 -> Convection/3(Cw_Tf)
  In Bus Element6/1 -> Convection/2(Cw_Tc)
  Bus Creator/1 -> QV/1
  Subsystem/2(QV_i_e) -> Bus Creator/1  "QV_i_e"
  Convection/1(QV_c_e) -> Bus Creator/2
  Convection/2(QV_i_c) -> Bus Creator/3
  Convection/3(QV_i_f) -> Bus Creator/4
  QV_i/1 -> Bus Creator/5  "QV_i"
  Subsystem/1(R_a) -> R_a/1
  Windows/1 -> Subsystem/4(Windows)
  Bus Selector1/1 -> Subsystem/3(<Tair>)  "<Tair>"
  In Bus Element3/1 -> Subsystem/2(wind_speed)
  In Bus Element2/1 -> Subsystem/1(T_e)
  In Bus Element/1 -> Convection/6(rho_i), Subsystem/5(rho_i)
  In Bus Element5/1 -> Convection/7(C_w)
  In Bus Element4/1 -> Convection/4(T_e)
  In Bus Element1/1 -> Convection/5(wind_speed)
  Convection/4(QP) -> QP/1
  Indoor Temperature/1 -> Convection/1(IndoorTemp), Bus Selector1/1

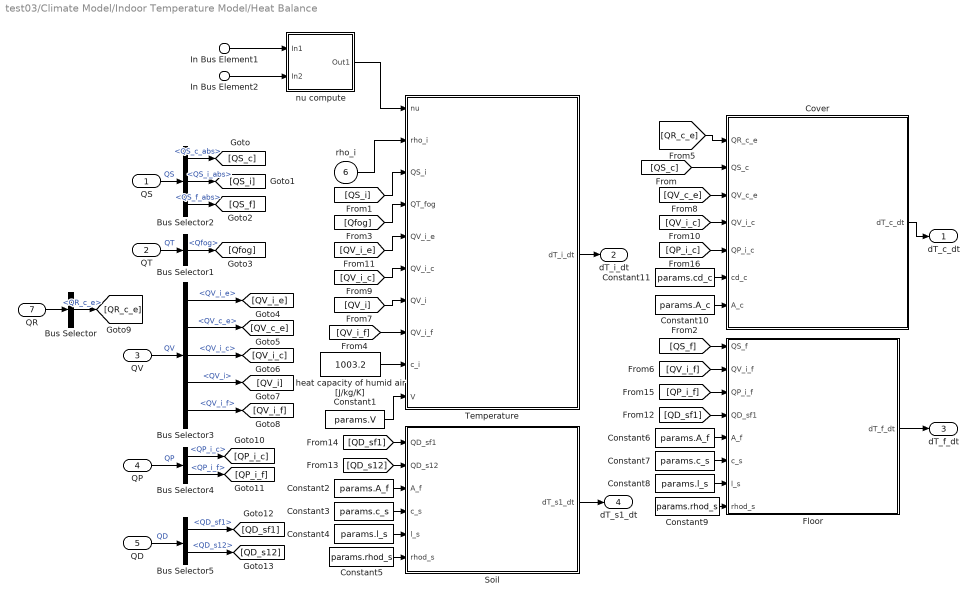
== system test03/Climate Model/Indoor Temperature Model/Heat Balance ==
  QS : Inport
  QT : Inport  Port=2
  QV : Inport  Port=3
  QP : Inport  Port=4
  QD : Inport  Port=5
  rho_i : Inport  Port=6
  QR : Inport  Port=7
  In Bus Element1 : Inport  Port=8  PortName=screen  Element=beta
  In Bus Element2 : Inport  Port=8  PortName=screen  Element=value
  " Cover" : MATLAB Function  TreatAsAtomicUnit=on
  " Floor" : MATLAB Function  TreatAsAtomicUnit=on
  " Soil" : MATLAB Function  TreatAsAtomicUnit=on
  " Temperature" : MATLAB Function  TreatAsAtomicUnit=on
  Bus Selector : BusSelector  OutputSignals=QR_c_e
  Bus Selector1 : BusSelector  OutputSignals=Qfog
  Bus Selector2 : BusSelector  OutputSignals=QS_c_abs,QS_i_abs,QS_f_abs
  Bus Selector3 : BusSelector  OutputSignals=QV_i_e,QV_c_e,QV_i_c,QV_i,QV_i_f
  Bus Selector4 : BusSelector  OutputSignals=QP_i_c,QP_i_f
  Bus Selector5 : BusSelector  OutputSignals=QD_sf1,QD_s12
  Constant1 : Constant  Value=params.V
  Constant10 : Constant  Value=params.A_c
  Constant11 : Constant  Value=params.cd_c
  Constant2 : Constant  Value=params.A_f
  Constant3 : Constant  Value=params.c_s
  Constant4 : Constant  Value=params.l_s
  Constant5 : Constant  Value=params.rhod_s
  Constant6 : Constant  Value=params.A_f
  Constant7 : Constant  Value=params.c_s
  Constant8 : Constant  Value=params.l_s
  Constant9 : Constant  Value=params.rhod_s
  "heat capacity of humid air [J/kg/K] " : Constant  Value=1003.2
  nu compute : Subsystem
  dT_c_dt : Outport
  dT_i_dt : Outport  Port=2
  dT_f_dt : Outport  Port=3
  dT_s1_dt : Outport  Port=4
  wires:
  [QR_c_e] -> " Cover"/1(QR_c_e)
  Bus Selector/1 -> [QR_c_e]  "<QR_c_e>"
  QR/1 -> Bus Selector/1
  Constant11/1 -> " Cover"/6(cd_c)
  Constant10/1 -> " Cover"/7(A_c)
  Constant9/1 -> " Floor"/8(rhod_s)
  Constant8/1 -> " Floor"/7(l_s)
  Constant7/1 -> " Floor"/6(c_s)
  Constant6/1 -> " Floor"/5(A_f)
  Constant5/1 -> " Soil"/6(rhod_s)
  Constant4/1 -> " Soil"/5(l_s)
  Constant3/1 -> " Soil"/4(c_s)
  Constant2/1 -> " Soil"/3(A_f)
  Constant1/1 -> " Temperature"/10(V)
  "heat capacity of humid air [J/kg/K] "/1 -> " Temperature"/9(c_i)
  [QP_i_c] -> " Cover"/5(QP_i_c)
  [QP_i_f] -> " Floor"/3(QP_i_f)
  [QD_sf1] -> " Soil"/1(QD_sf1)
  [QD_s12] -> " Soil"/2(QD_s12)
  [QD_sf1] -> " Floor"/4(QD_sf1)
  Bus Selector5/2 -> [QD_s12]  "<QD_s12>"
  Bus Selector5/1 -> [QD_sf1]  "<QD_sf1>"
  Bus Selector4/2 -> [QP_i_f]  "<QP_i_f>"
  Bus Selector4/1 -> [QP_i_c]  "<QP_i_c>"
  [QV_i_e] -> " Temperature"/5(QV_i_e)
  [QV_i_c] -> " Cover"/4(QV_i_c)
  [QV_i_c] -> " Temperature"/6(QV_i_c)
  [QV_c_e] -> " Cover"/3(QV_c_e)
  [QV_i] -> " Temperature"/7(QV_i)
  [QV_i_f] -> " Floor"/2(QV_i_f)
  [QV_i_f] -> " Temperature"/8(QV_i_f)
  Bus Selector3/2 -> [QV_c_e]  "<QV_c_e>"
  Bus Selector3/3 -> [QV_i_c]  "<QV_i_c>"
  Bus Selector3/4 -> [QV_i]  "<QV_i>"
  Bus Selector3/5 -> [QV_i_f]  "<QV_i_f>"
  Bus Selector3/1 -> [QV_i_e]  "<QV_i_e>"
  [Qfog] -> " Temperature"/4(QT_fog)
  Bus Selector1/1 -> [Qfog]  "<Qfog>"
  [QS_f] -> " Floor"/1(QS_f)
  [QS_i] -> " Temperature"/3(QS_i)
  [QS_c] -> " Cover"/2(QS_c)
  Bus Selector2/3 -> [QS_f]  "<QS_f_abs>"
  Bus Selector2/2 -> [QS_i]  "<QS_i_abs>"
  Bus Selector2/1 -> [QS_c]  "<QS_c_abs>"
  " Cover"/1(dT_c_dt) -> dT_c_dt/1
  QV/1 -> Bus Selector3/1  "QV"
  rho_i/1 -> " Temperature"/2(rho_i)
  QP/1 -> Bus Selector4/1  "QP"
  QS/1 -> Bus Selector2/1  "QS"
  QT/1 -> Bus Selector1/1  "QT"
  " Temperature"/1(dT_i_dt) -> dT_i_dt/1
  QD/1 -> Bus Selector5/1  "QD"
  " Soil"/1(dT_s1_dt) -> dT_s1_dt/1
  " Floor"/1(dT_f_dt) -> dT_f_dt/1
  In Bus Element1/1 -> nu compute/1(In1)
  In Bus Element2/1 -> nu compute/2(In2)
  nu compute/1(Out1) -> " Temperature"/1(nu)

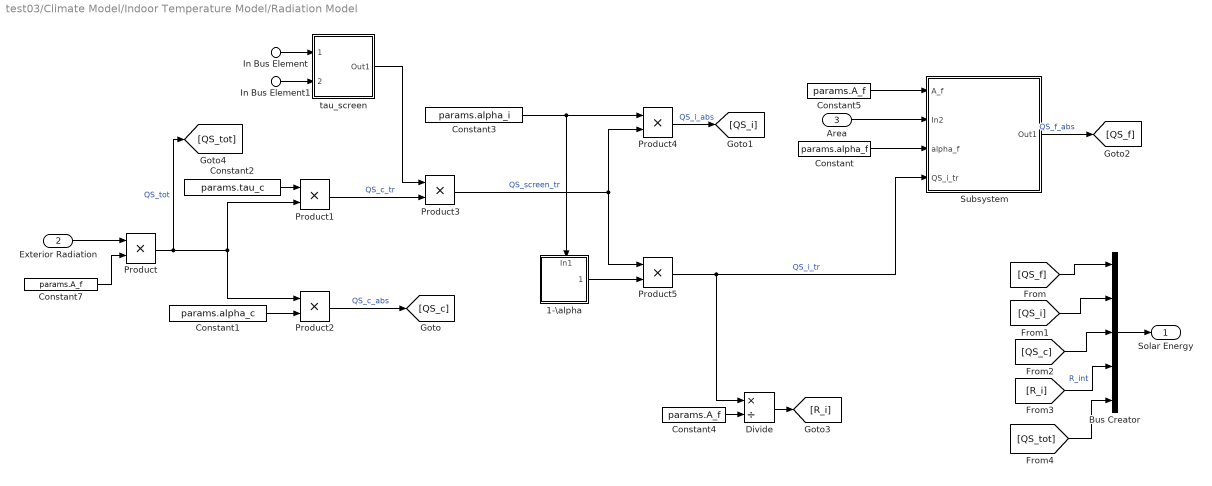
== system test03/Climate Model/Indoor Temperature Model/Radiation Model ==
  In Bus Element : Inport  PortName=screen  Element=gamma_max
  In Bus Element1 : Inport  PortName=screen  Element=value
  Exterior Radiation : Inport  Port=2
  Area : Inport  Port=3
  1-\alpha : Subsystem
      settings: PortSchema="{\"entries\":[{\"content\":{\"sides\":[{\"content\":{\"connectorIds\":[]},\"type\":\"ConnectorPlacement.EquallySpacedRectSide\",\"uuid\":\"bf116baa-1c91-42ba-b5ce-6949a5122443\"},{\"content\":{\"connectorIds\":[\"Out1\"],\"side\":\"RIGHT\"},\"type\":\"ConnectorPlacement.EquallySpacedRectSide\",\"uuid\":\"479b2a41-aae8-4d0f-95ce-40d0c52850dd\"},{\"content\":{\"connectorIds\":[\"In1\"],\"side\":\"TOP\"},\"type\":\"ConnectorPlacement.EquallySpacedRectSide\",\"uuid\":\"d0364cd7-422a-4274-8084-cbaa88b34f4b\"}]},\"type\":\"ConnectorPlacement.EquallySpacedConnector\",\"uuid\":\"3d8ba820-72ed-4082-b0d9-d7ce7398093f\"}],\"packageUris\":[\"http://schema.mathworks.com/mf0/Connector/R2020b\"],\"version\":\"1.0\"}"
  Bus Creator : BusCreator  Inputs=5
  Constant : Constant  Value=params.alpha_f
  Constant1 : Constant  Value=params.alpha_c
  Constant2 : Constant  Value=params.tau_c
  Constant3 : Constant  Value=params.alpha_i
  Constant4 : Constant  Value=params.A_f
  Constant5 : Constant  Value=params.A_f
  Constant7 : Constant  Value=params.A_f
  Divide : Product  Inputs=*/
  Product{,1..5} (6 alike) : Product
  Subsystem : Subsystem
  tau_screen : Subsystem
  "Solar Energy  " : Outport
  wires:
  Divide/1 -> [R_i]
  Constant4/1 -> Divide/2
  Subsystem/1(Out1) -> [QS_f]  "QS_f_abs"
  Product5/1 -> Divide/1, Subsystem/4(QS_i_tr)  "QS_i_tr"
  Constant/1 -> Subsystem/3(alpha_f)
  Area/1 -> Subsystem/2(In2)
  Constant5/1 -> Subsystem/1(A_f)
  Product4/1 -> [QS_i]  "QS_i_abs"
  1-\alpha/1(Out1) -> Product5/2
  Constant3/1 -> 1-\alpha/1(In1), Product4/1
  Product3/1 -> Product5/1, Product4/2  "QS_screen_tr"
  tau_screen/1(Out1) -> Product3/1
  Product2/1 -> [QS_c]  "QS_c_abs"
  Product1/1 -> Product3/2  "QS_c_tr"
  Constant1/1 -> Product2/2
  Constant2/1 -> Product1/1
  Product/1 -> [QS_tot], Product1/2, Product2/1  "QS_tot"
  Constant7/1 -> Product/2
  Exterior Radiation/1 -> Product/1
  [R_i] -> Bus Creator/4  "R_int"
  [QS_c] -> Bus Creator/3
  Bus Creator/1 -> "Solar Energy  "/1
  [QS_f] -> Bus Creator/1
  [QS_i] -> Bus Creator/2
  [QS_tot] -> Bus Creator/5
  In Bus Element1/1 -> tau_screen/2(screen)
  In Bus Element/1 -> tau_screen/1(gamma)

== system test03/Climate Model/Indoor Temperature Model/Subsystem ==
  Tc : Inport
  Te : Inport  Port=2
  " Stefan-Boltzmann constant [W/m^2/K^4] " : Constant  Value=5.67e-8
  Bus Creator : BusCreator  Inputs=1
  Constant : Constant  Value=4
  Constant1 : Constant  Value=4
  Constant2 : Constant  Value=params.A_c
  Minus : Sum  Inputs=+-
  Product : Product  Inputs=4
  Square : Math  Operator=pow  SaturateOnIntegerOverflow=on
  Square1 : Math  Operator=pow  SaturateOnIntegerOverflow=on
  k : Constant  Value=0.985
  QR : Outport
  wires:
  Bus Creator/1 -> QR/1
  Product/1 -> Bus Creator/1  "QR_c_e"
  Constant1/1 -> Square1/2
  " Stefan-Boltzmann constant [W/m^2/K^4] "/1 -> Product/4
  k/1 -> Product/3
  Minus/1 -> Product/1
  Constant2/1 -> Product/2
  Square1/1 -> Minus/2
  Square/1 -> Minus/1
  Te/1 -> Square1/1
  Constant/1 -> Square/2
  Tc/1 -> Square/1

== system test03/Climate Model/Gases Exchange/Carbon Dynamics/Carbon Exchange Indoor-Outdoor ==
  R_a : Inport
  C_c : Inport  Port=2
  C_ce : Inport  Port=3
  Minus : Sum  Inputs=+-
  Product : Product
  MC_i_e : Outport
  wires:
  Product/1 -> MC_i_e/1
  R_a/1 -> Product/1
  Minus/1 -> Product/2
  C_ce/1 -> Minus/2
  C_c/1 -> Minus/1

== system test03/Climate Model/Gases Exchange/Carbon Dynamics/External CO2 Concentration ==
  T_e : Inport
  Divide : Product  Inputs=**//
  Gain : Gain  Gain=4e-4
  M_c : Constant  Value=0.0440
  R : Constant  Value=8.3140
  atm : Constant  Value=101300
  C_ce : Outport
  wires:
  Gain/1 -> C_ce/1
  Divide/1 -> Gain/1
  T_e/1 -> Divide/4
  M_c/1 -> Divide/2
  R/1 -> Divide/3
  atm/1 -> Divide/1

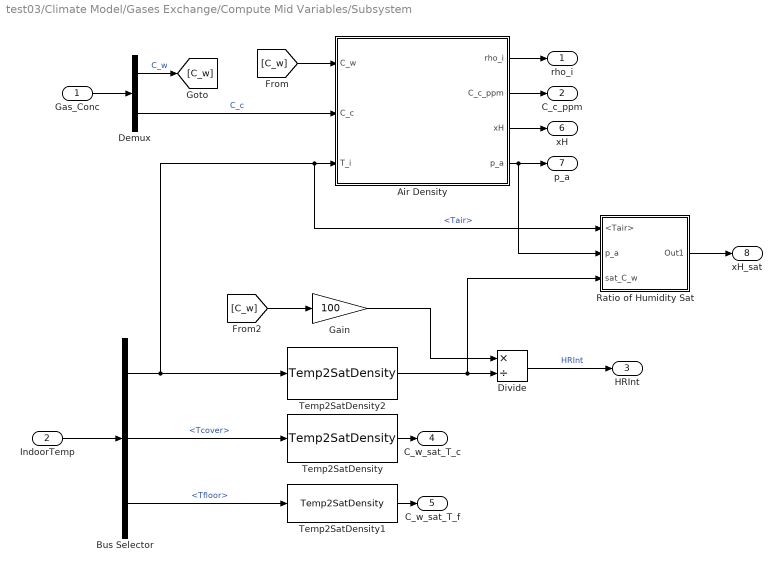
== system test03/Climate Model/Gases Exchange/Compute Mid Variables/Subsystem ==
  Gas_Conc : Inport
  IndoorTemp : Inport  Port=2
  Air Density : MATLAB Function  TreatAsAtomicUnit=on
  Bus Selector : BusSelector  OutputSignals=Tair,Tcover,Tfloor
  Demux : Demux  Outputs=2
  Divide : Product  Inputs=*/
  Gain : Gain  Gain=100
  Ratio of Humidity Sat : Subsystem
  Temp2SatDensity : HORTISIM/Other  Functions/Temp2SatDensity  SystemSampleTime=-1  VariantActivationTime=update diagram  Latency=0  AutoFrameSizeCalculation=off
      settings: SourceProductName=Horti Simulator
  Temp2SatDensity1 : HORTISIM/Other  Functions/Temp2SatDensity  SystemSampleTime=-1  VariantActivationTime=update diagram  Latency=0  AutoFrameSizeCalculation=off
      settings: SourceProductName=Horti Simulator
  Temp2SatDensity2 : HORTISIM/Other  Functions/Temp2SatDensity  SystemSampleTime=-1  VariantActivationTime=update diagram  Latency=0  AutoFrameSizeCalculation=off
      settings: SourceProductName=Horti Simulator
  rho_i : Outport
  C_c_ppm : Outport  Port=2
  HRInt : Outport  Port=3
  C_w_sat_T_c : Outport  Port=4
  C_w_sat_T_f : Outport  Port=5
  xH : Outport  Port=6
  p_a : Outport  Port=7
  xH_sat : Outport  Port=8
  wires:
  Ratio of Humidity Sat/1(Out1) -> xH_sat/1
  Divide/1 -> HRInt/1  "HRInt"
  [C_w] -> Gain/1
  Gain/1 -> Divide/1
  Temp2SatDensity2/1 -> Divide/2, Ratio of Humidity Sat/3(sat_C_w)
  Air Density/4(p_a) -> p_a/1, Ratio of Humidity Sat/2(p_a)
  Air Density/3(xH) -> xH/1
  [C_w] -> Air Density/1(C_w)
  Air Density/2(C_c_ppm) -> C_c_ppm/1
  Air Density/1(rho_i) -> rho_i/1
  Demux/2 -> Air Density/2(C_c)  "C_c"
  Demux/1 -> [C_w]  "C_w"
  Temp2SatDensity1/1 -> C_w_sat_T_f/1
  Temp2SatDensity/1 -> C_w_sat_T_c/1
  Bus Selector/3 -> Temp2SatDensity1/1  "<Tfloor>"
  Bus Selector/2 -> Temp2SatDensity/1  "<Tcover>"
  Gas_Conc/1 -> Demux/1
  Bus Selector/1 -> Temp2SatDensity2/1, Air Density/3(T_i), Ratio of Humidity Sat/1(<Tair>)  "<Tair>"
  IndoorTemp/1 -> Bus Selector/1

== system test03/Climate Model/Gases Exchange/Water Dynamics/Subsystem ==
  <Temperature> : Inport
  <Exterior Humidity> : Inport  Port=2
  Gain : Gain  Gain=1/100
  Product : Product
  Temp2SatDensity : HORTISIM/Other  Functions/Temp2SatDensity  SystemSampleTime=-1  VariantActivationTime=update diagram  Latency=0  AutoFrameSizeCalculation=off
      settings: SourceProductName=Horti Simulator
  C_w_Te : Outport
  wires:
  Gain/1 -> Product/2
  Temp2SatDensity/1 -> Product/1  "C_w_sat_Te"
  <Exterior Humidity>/1 -> Gain/1
  <Temperature>/1 -> Temp2SatDensity/1
  Product/1 -> C_w_Te/1  "C_w_Te"

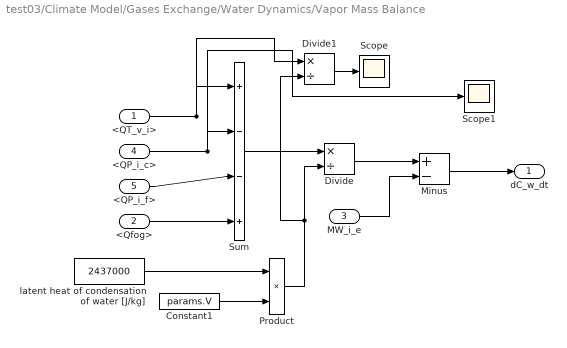
== system test03/Climate Model/Gases Exchange/Water Dynamics/Vapor Mass Balance ==
  <QT_v_i> : Inport
  <Qfog> : Inport  Port=2
  MW_i_e : Inport  Port=3
  <QP_i_c> : Inport  Port=4
  <QP_i_f> : Inport  Port=5
  Constant1 : Constant  Value=params.V
  Divide : Product  Inputs=*/
  Divide1 : Product  Inputs=*/
  Minus : Sum  Inputs=+-
  Product : Product
  Scope : Scope
  Scope1 : Scope
  Sum : Sum  Inputs=|+--+
  latent heat of condensation of water [J/kg] : Constant  Value=2437000
  dC_w_dt : Outport
  wires:
  Divide1/1 -> Scope/1
  Minus/1 -> dC_w_dt/1
  MW_i_e/1 -> Minus/2
  Divide/1 -> Minus/1
  Product/1 -> Divide/2, Divide1/2
  Sum/1 -> Divide/1
  <Qfog>/1 -> Sum/4
  <QP_i_f>/1 -> Sum/3
  <QP_i_c>/1 -> Sum/2, Scope1/1
  <QT_v_i>/1 -> Sum/1, Divide1/1
  Constant1/1 -> Product/2
  latent heat of condensation of water [J/kg]/1 -> Product/1

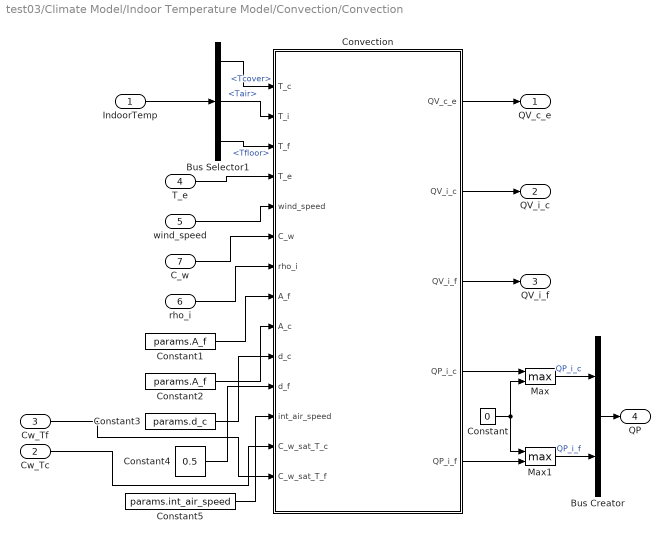
== system test03/Climate Model/Indoor Temperature Model/Convection/Convection ==
  IndoorTemp : Inport
  Cw_Tc : Inport  Port=2
  Cw_Tf : Inport  Port=3
  T_e : Inport  Port=4
  wind_speed : Inport  Port=5
  rho_i : Inport  Port=6
  C_w : Inport  Port=7
  Bus Creator : BusCreator  Inputs=2
  Bus Selector1 : BusSelector  OutputSignals=Tcover,Tair,Tfloor
  Constant : Constant  Value=0
  Constant1 : Constant  Value=params.A_f
  Constant2 : Constant  Value=params.A_f
  Constant3 : Constant  Value=params.d_c
  Constant4 : Constant  Value=0.5
  Constant5 : Constant  Value=params.int_air_speed
  Convection : MATLAB Function  TreatAsAtomicUnit=on
  Max : MinMax  Function=max  Inputs=2
  Max1 : MinMax  Function=max  Inputs=2
  QV_c_e : Outport
  QV_i_c : Outport  Port=2
  QV_i_f : Outport  Port=3
  QP : Outport  Port=4
  wires:
  Cw_Tc/1 -> Convection/13(C_w_sat_T_c)
  Cw_Tf/1 -> Convection/14(C_w_sat_T_f)
  Constant5/1 -> Convection/12(int_air_speed)
  Constant4/1 -> Convection/11(d_f)
  Constant3/1 -> Convection/10(d_c)
  Constant2/1 -> Convection/9(A_c)
  Constant1/1 -> Convection/8(A_f)
  wind_speed/1 -> Convection/5(wind_speed)
  T_e/1 -> Convection/4(T_e)
  Bus Selector1/3 -> Convection/3(T_f)  "<Tfloor>"
  Bus Selector1/2 -> Convection/2(T_i)  "<Tair>"
  Bus Selector1/1 -> Convection/1(T_c)  "<Tcover>"
  IndoorTemp/1 -> Bus Selector1/1
  Max/1 -> Bus Creator/1  "QP_i_c"
  Max1/1 -> Bus Creator/2  "QP_i_f"
  Convection/4(QP_i_c) -> Max/1
  Convection/5(QP_i_f) -> Max1/2
  Constant/1 -> Max/2, Max1/1
  rho_i/1 -> Convection/7(rho_i)
  C_w/1 -> Convection/6(C_w)
  Bus Creator/1 -> QP/1
  Convection/3(QV_i_f) -> QV_i_f/1
  Convection/2(QV_i_c) -> QV_i_c/1
  Convection/1(QV_c_e) -> QV_c_e/1

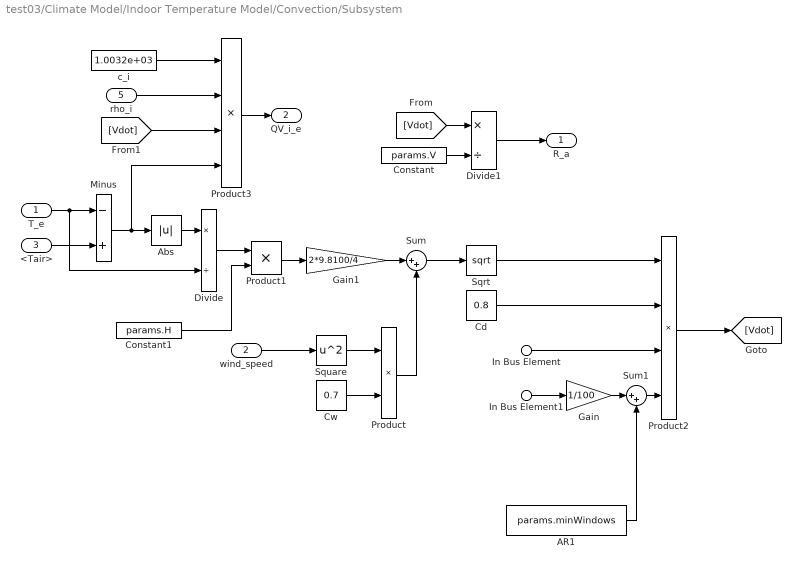
== system test03/Climate Model/Indoor Temperature Model/Convection/Subsystem ==
  T_e : Inport
  wind_speed : Inport  Port=2
  <Tair> : Inport  Port=3
  In Bus Element1 : Inport  Port=4  PortName=Windows  Element=value
  In Bus Element : Inport  Port=4  PortName=Windows  Element=AR
  rho_i : Inport  Port=5
  AR1 : Constant  Value=params.minWindows  VectorParams1D=off
  Abs : Abs
  Cd : Constant  Value=0.8  VectorParams1D=off
  Constant : Constant  Value=params.V
  Constant1 : Constant  Value=params.H
  Cw : Constant  Value=0.7  VectorParams1D=off
  Divide : Product  Inputs=*/
  Divide1 : Product  Inputs=*/
  Gain : Gain  Gain=1/100
  Gain1 : Gain  Gain=2*9.8100/4
  Minus : Sum  Inputs=-+
  Product : Product
  Product1 : Product
  Product2 : Product  Inputs=4
  Product3 : Product  Inputs=4
  Sqrt : Sqrt  SaturateOnIntegerOverflow=on
  Square : Math  Operator=square  SaturateOnIntegerOverflow=on
  Sum : Sum  Inputs=|++
  Sum1 : Sum  Inputs=|++
  c_i : Constant  Value=1.0032e+03  VectorParams1D=off
  R_a : Outport
  QV_i_e : Outport  Port=2
  wires:
  AR1/1 -> Sum1/2
  Sum1/1 -> Product2/4
  Gain/1 -> Sum1/1
  Product3/1 -> QV_i_e/1
  c_i/1 -> Product3/1
  rho_i/1 -> Product3/2
  [Vdot] -> Product3/3
  Divide1/1 -> R_a/1
  Constant/1 -> Divide1/2
  [Vdot] -> Divide1/1
  Product2/1 -> [Vdot]
  Cd/1 -> Product2/2
  Sqrt/1 -> Product2/1
  Sum/1 -> Sqrt/1
  Gain1/1 -> Sum/1
  Product1/1 -> Gain1/1
  Divide/1 -> Product1/1
  Constant1/1 -> Product1/2
  Abs/1 -> Divide/1
  Minus/1 -> Abs/1, Product3/4
  <Tair>/1 -> Minus/2
  T_e/1 -> Divide/2, Minus/1
  Product/1 -> Sum/2
  Cw/1 -> Product/2
  Square/1 -> Product/1
  wind_speed/1 -> Square/1
  In Bus Element1/1 -> Gain/1
  In Bus Element/1 -> Product2/3

== system test03/Climate Model/Indoor Temperature Model/Heat Balance/nu compute ==
  In1 : Inport
  In2 : Inport  Port=2
  Constant : Constant
  Gain : Gain  Gain=1/100
  Product : Product
  Scope : Scope
  Sum : Sum  Inputs=|++
  Out1 : Outport
  wires:
  Sum/1 -> Scope/1, Out1/1
  In1/1 -> Product/1
  Constant/1 -> Sum/2
  In2/1 -> Gain/1
  Product/1 -> Sum/1
  Gain/1 -> Product/2

== system test03/Climate Model/Indoor Temperature Model/Radiation Model/1-\alpha ==
  In1 : Inport
  Constant6 : Constant
  Minus : Sum  Inputs=+-
  Out1 : Outport
  wires:
  Constant6/1 -> Minus/1
  In1/1 -> Minus/2
  Minus/1 -> Out1/1

== system test03/Climate Model/Indoor Temperature Model/Radiation Model/Subsystem ==
  A_f : Inport
  In2 : Inport  Port=2
  alpha_f : Inport  Port=3
  QS_i_tr : Inport  Port=4
  Divide : Product  Inputs=*/**
  Minus : Sum  Inputs=+-
  Out1 : Outport
  wires:
  Minus/1 -> Divide/1
  alpha_f/1 -> Divide/3
  In2/1 -> Minus/2
  Divide/1 -> Out1/1
  A_f/1 -> Minus/1, Divide/2
  QS_i_tr/1 -> Divide/4

== system test03/Climate Model/Indoor Temperature Model/Radiation Model/tau_screen ==
  gamma : Inport
  screen : Inport  Port=2
  Constant3 : Constant
  Divide : Product  Inputs=**
  Gain : Gain  Gain=1/100
  Minus : Sum  Inputs=+-
  Out1 : Outport
  wires:
  Constant3/1 -> Minus/1
  screen/1 -> Divide/2
  Minus/1 -> Out1/1
  Gain/1 -> Minus/2
  Divide/1 -> Gain/1
  gamma/1 -> Divide/1

== system test03/Climate Model/Gases Exchange/Compute Mid Variables/Subsystem/Ratio of Humidity Sat ==
  <Tair> : Inport
  p_a : Inport  Port=2
  sat_C_w : Inport  Port=3
  " molar mass of water [kg/mol]" : Constant  Value=0.0180
  Divide1 : Product  Inputs=*/
  Divide2 : Product  Inputs=*/
  Gain1 : Gain  Gain=0.62198
  Minus : Sum  Inputs=+-
  Product : Product  Inputs=3
  gas constant [J/mol/K] : Constant  Value=8.3140
  Out1 : Outport
  wires:
  Divide2/1 -> Gain1/1
  Divide1/1 -> Minus/2, Divide2/1  "p_w^*"
  gas constant [J/mol/K]/1 -> Product/2
  " molar mass of water [kg/mol]"/1 -> Divide1/2
  Product/1 -> Divide1/1
  <Tair>/1 -> Product/1
  sat_C_w/1 -> Product/3
  Gain1/1 -> Out1/1
  Minus/1 -> Divide2/2
  p_a/1 -> Minus/1

== matlab function test03/Climate Model/Indoor Temperature Model/Conduction/Conduction ==
  data: T_f input; T_s1 input; QD_sf1 output; QD_s12 output; A_f input; lam_s input; l_s input; T_ss input
function [QD_sf1,QD_s12] = fcn(T_f,T_s1,A_f,lam_s,l_s,T_ss)

%
%%
% GEOMETRY
% ========
% A_f = p.A_f; % greenhouse floor area [m^2]
% 
% % FLOOR 
% % =====================
% lam_s= p.lam_s; %thermal conductivity of soil layers [W/mK] Concrete, Soil, Clay
% l_s  = p.l_s; %thickness of soil layers [m]
% 
% T_ss = p.T_ss; %deep soil temperature [K]

%%      Conduction
% Floor layers 
% 
QD_sf1 = A_f*lam_s(1)/l_s(1).*(T_f - T_s1); 
QD_s12 = A_f*lam_s(2)/l_s(2).*(T_s1 - T_ss);

== matlab function test03/Climate Model/Indoor Temperature Model/Convection/Convection/Convection ==
  data: QV_c_e output; QV_i_c output; QV_i_f output; T_c input; T_i input; T_f input; T_e input; wind_speed input; QP_i_c output; QP_i_f output; C_w input; rho_i input; A_f input; A_c input; d_c input; d_f input; int_air_speed input; C_w_sat_T_c input; C_w_sat_T_f input
function [QV_c_e,QV_i_c,QV_i_f,QP_i_c,QP_i_f] = fcn( T_c,T_i,T_f,T_e,wind_speed,C_w,rho_i,A_f,A_c,d_c,d_f,int_air_speed,C_w_sat_T_c,C_w_sat_T_f)

% CONSTANTS
% =========
g = 9.8100; % acceleration due to gravity [m/s^2]
lambda = 0.0250; % thermal conductivity of air [W/m/K]

Le = 0.8190; % Lewis number [-] 
nu =  1.5100e-05; % kinematic viscosity [m^2/s]

%%
c_i = 1.0032e+03;
H_fg = 2437000;

%%

if wind_speed<0
    wind_speed = 0;
end
%%      Convection

% The Grashof and Reynolds numbers are calculated, and then the Nusselt
% number calculated as the larger of the 'free' Nusselt number, based on
% the Grashof number, and the 'forced' Nusselt number, based on the
% Reynolds number. The heat transferred per unit time is then calculated
% based on this. The first subscript is where heat is transferred from, and
% the second subscript where heat is transferred to.

% Cover to external air
Gr = g*d_c^3/(T_e*nu^2)*abs(T_c - T_e);
Re = wind_speed*d_c/nu;
Nu = lamorturb(Gr, Re);
QV_c_e = A_c.*Nu*lambda.*(T_c - T_e)/d_c;

% Internal air to cover
Gr = g*d_c^3./(T_i*nu^2).*abs(T_i - T_c);
Re = int_air_speed*d_c/nu;  
[Nu, Sh] = lamorturb(Gr, Re, Le);
QV_i_c = A_c.*Nu*lambda.*(T_i - T_c)/d_c;
QP_i_c = A_c*H_fg./(rho_i*c_i).*Sh/Le*lambda/d_c.*(C_w - C_w_sat_T_c);
%QP_i_c = max(QP_i_c,0); % assumed no evaporation from the cover, only condensation

%Internal air to floor
Gr = g*d_f^3./(T_i*nu^2).*abs(T_i - T_f); 
Re = int_air_speed*d_f/nu;
[Nu, Sh] = lamorturb(Gr, Re, Le);
QV_i_f = A_f.*Nu*lambda.*(T_i - T_f)/d_f;
QP_i_f = A_f*H_fg./(rho_i*c_i).*Sh/Le*lambda/d_f.*(C_w - C_w_sat_T_f); 
%QP_i_f = max(QP_i_f,0); % assumed no evaporation from the floor, only condensation

== matlab function test03/Climate Model/Indoor Temperature Model/Heat Balance/ Soil ==
  data: QD_sf1 input; QD_s12 input; dT_s1_dt output; A_f input; c_s input; l_s input; rhod_s input
function dT_s1_dt  = fcn(QD_sf1,QD_s12,A_f,c_s,l_s,rhod_s)



%% Soil 1
c_Ts1 = 1./(rhod_s(2) * c_s(2) * l_s(2)*A_f);
%
dT_s1_dt = c_Ts1*(QD_sf1 - QD_s12);
%%

== matlab function test03/Climate Model/Indoor Temperature Model/Heat Balance/ Cover ==
  data: QR_c_e input; QS_c input; QV_c_e input; QV_i_c input; QP_i_c input; dT_c_dt output; cd_c input; A_c input
function dT_c_dt = fcn(QR_c_e, QS_c,QV_c_e,QV_i_c,QP_i_c,cd_c,A_c)

%% Cover Temperature
dT_c_dt = 1./(A_c*cd_c).*(+QV_i_c   - QV_c_e  + QS_c + QP_i_c - QR_c_e);

== matlab function test03/Climate Model/Indoor Temperature Model/Heat Balance/ Floor ==
  data: QS_f input; QV_i_f input; QP_i_f input; QD_sf1 input; dT_f_dt output; A_f input; c_s input; l_s input; rhod_s input
function dT_f_dt  = fcn(QS_f,QV_i_f,QP_i_f,QD_sf1,A_f,c_s,l_s,rhod_s)



%% Floor
c_Tf =  1./(rhod_s(1) * A_f * c_s(1) * l_s(1));
%
dT_f_dt  =c_Tf*(QV_i_f  + QS_f - QD_sf1 + QP_i_f);

== matlab function test03/Climate Model/Gases Exchange/Compute Mid Variables/Subsystem/Air Density ==
  data: C_w input; C_c input; T_i input; rho_i output; C_c_ppm output; xH output; p_a output
function [rho_i,C_c_ppm,xH,p_a] =   Air(C_w,C_c,T_i)

% CONSTANTS
% =========  
atm = 101300; % standard atmospheric pressure [Pa]
M_a = 0.0290; % molar mass of dry air [kg/mol]                                                                 
R   = 8.3140; % gas constant [J/mol/K]
M_w = 0.0180; % molar mass of water [kg/mol]
M_c = 0.0440; % molar mass of CO2 [kg/mol]


%%
p_w = C_w*R.*T_i/M_w; % Partial pressure of water [Pa]
p_a = (atm - p_w);
rho_i  = (p_a*M_a + p_w*M_w)./(R*T_i); % Density of air [kg/m^3]
C_c_ppm = C_c*R.*T_i/(M_c*atm)*1e6; % CO2 concentration in ppm

xH = 0.62198* p_w /(p_a - p_w);
%%

== matlab function test03/Climate Model/Indoor Temperature Model/Heat Balance/ Temperature ==
  data: nu input; rho_i input; QS_i input; QT_fog input; QV_i_e input; QV_i_c input; QV_i input; QV_i_f input; dT_i_dt output; c_i input; V input
function dT_i_dt  = fcn( nu, rho_i ,QS_i,QT_fog,QV_i_e,QV_i_c,QV_i,QV_i_f,c_i,V)


%% Air Temperature

c_Ti = 1./(nu*V.*rho_i*c_i);

dT_i_dt = c_Ti*(  QV_i - QV_i_f - QV_i_c - QV_i_e + QS_i  - QT_fog); 
%%
